simulink model "Form_Finding_Simulink"  (R2022a)
settings: Solver=ode14x  StartTime=0.0  StopTime=0.2  FixedStep=0.00005  RelTol=1e-3
values from neighbouring files (symbols this model uses):
  a_joint = 160/180*pi    (= 2.79252680319)    [Form_Finding_Activation.m]
  F_motor = F    (= 0)    [Form_Finding_Activation.m]
  g = [0;0;-9.81]    [Form_Finding_Activation.m]
  k_cable = 1200    [Form_Finding_Activation.m]
  k_joint = 35    [Form_Finding_Activation.m]
  l_cable = sqrt(6)/4*l_leg*sin(a_joint/2)*(1 - delta)    [Form_Finding_Activation.m]
  m_bar = density*(l_leg*pi*0.005^2)+ m_motor + m_battery    (= 0.662767695314)    [Form_Finding_Activation.m]
  x10_ini = x4_ini+[0 -2*bent_bar 0]    [Form_Finding_Activation.m]
  x11_ini = 2*bent_bar*rotVec([1 0 0],[0 1 0],-90-theta) + x5_ini    [Form_Finding_Activation.m]
  x12_ini = 2*bent_bar*rotVec([1 0 0],[0 1 0],-theta) + x6_ini    [Form_Finding_Activation.m]
  x1_ini = [0 0 0]    [Form_Finding_Activation.m]
  x2_ini = bent_bar*rotVec([1 0 0],[0 1 0],-theta)+ 0.5*sep*rotVec([1 0 0],[0 1 0],90-theta) + [0 sep/2 0]    [Form_Finding_Activation.m]
  x3_ini = [d6x   -sep/2         0]    [Form_Finding_Activation.m]
  x4_ini = bent_bar*rotVec([1 0 0],[0 1 0],-theta) + 0.5*sep*rotVec([1 0 0],[0 1 0],-90-theta) + [0 sep/2 0]    [Form_Finding_Activation.m]
  x5_ini = sep*rotVec([1 0 0],[0 1 0],-theta) + x3_ini    [Form_Finding_Activation.m]
  x6_ini = [0 -sep 0]    [Form_Finding_Activation.m]
  x7_ini = 2*bent_bar*rotVec([1 0 0],[0 1 0],-theta) + x1_ini    [Form_Finding_Activation.m]
  x8_ini = x2_ini + [0 -2*bent_bar 0]    [Form_Finding_Activation.m]
  x9_ini = 2*bent_bar*rotVec([1 0 0],[0 1 0],-90-theta) + x3_ini    [Form_Finding_Activation.m]
undefined symbols (not defined in the file or in its folder): l_bar
(part 2 of 2)

== matlab function Form_Finding_Simulink/6 joints/Joint bar 6--12 ==
  data: xi input; alpha output; xj input; xk input; l input; x_joint output
function [alpha, x_joint]  = angle(xi, xj, xk, l)
%% Calculating the angle
d = norm(xi - xj); % Nodal distance
mag = (l^2-2*d^2)/l^2; % Term inside the inverse cosine to calculate the angle
alpha = acos(mag); % Angle of the joint

%% Plotting the Joint
% Distance from axis
d = l/2*cos(alpha/2);

% Vectors used for determination of the normal vector
nxi = transpose(xi);
nxj = transpose(xj);
nxk = transpose(xk);

% Normal vector of a plane created by a set of 2 parallel bars
normal = cross(nxi-nxj, nxi-nxk);
N = normal/norm(normal);

% Vector along the line between bar-connected nodes
x = nxj - nxi;
X = x/norm(x);

% Vector pointing outwards 
V = rotVec(X,N,-90);

% Position vector of the joint, to be used for plotting
x_joint = transpose(d*V + (nxj+nxi)/2);

end

== matlab function Form_Finding_Simulink/24 cables/cable 1--4 ==
  data: out_i output; E_cable output; out_j output; k_cable input; l_cable input; xi input; xj input
function [out_i, E_cable, out_j]= cable(k_cable, l_cable,xi,xj)
% Node distance
dist = norm(xi-xj);

% Difference of node distance with the cable rest length
D = dist-l_cable;

% If the cable is in tension, then the force is calculated. When the cable is slack, the force is zero 
if  dist-l_cable >= 0
    D = dist-l_cable;
elseif dist-l_cable < 0
    D = 0;
end

% Forces on end nodes
out_i = k_cable*D*(xj-xi)/dist;
out_j = -k_cable*D*(xj-xi)/dist;

% Potential energy stored in the cable
E_cable = 0.5*k_cable*D^2;
end

== matlab function Form_Finding_Simulink/6 joints/Force bar 6--12 ==
  data: T input; xi input; xj input; m input; torsion_i output; torsion_j output; k_joint input; alpha input; l_bar input; a_joint input; g input
function [torsion_i, torsion_j]= Force(T, xi, xj, m, k_joint, alpha, l_bar, a_joint, g)
% Node distance
dist = norm(xj-xi);

% Force exerted by the joint at the end node. The force is zero when the
% deflection angle is larger than a_joint
if alpha < a_joint
    F_torsion = 1/2 * k_joint * (a_joint - alpha) / (cos(alpha/2)*l_bar/2);
else
    F_torsion = 0;
end

% Gravitational force:
Fg_j = m*g/2;

% Motor Force, also with the lever effect incorporated
F_motor = T/(l_bar*cos(alpha/2));

% Calculation of the two parts of the torsion
torsion_i = (F_torsion - F_motor) *(xi-xj)/dist; % % No gravity on this node because it is on the ground
torsion_j = (F_torsion - F_motor) *(xj-xi)/dist + Fg_j;

end

== matlab function Form_Finding_Simulink/12 nodes /node  4/MATLAB Function ==
  data: X input; F_out output; F_in input
function F_out = ground_constraint(X,F_in)
if X(3) <= 0 && F_in(3) < 0 
    F_out = [F_in(1);F_in(2);0];
else
    F_out = F_in;
end
end

== matlab function Form_Finding_Simulink/12 nodes /node  7/MATLAB Function ==
  data: X input; F_out output; F_in input
function F_out = ground_constraint(X,F_in)
if X(3) <= 0 && F_in(3) < 0 
    F_out = [F_in(1);F_in(2);0];
else
    F_out = F_in;
end
end

== matlab function Form_Finding_Simulink/12 nodes /node  8/MATLAB Function ==
  data: X input; F_out output; F_in input
function F_out = ground_constraint(X,F_in)
if X(3) <= 0 && F_in(3) < 0 
    F_out = [F_in(1);F_in(2);0];
else
    F_out = F_in;
end

end

== matlab function Form_Finding_Simulink/12 nodes /node  9/MATLAB Function ==
  data: X input; F_out output; F_in input
function F_out = ground_constraint(X,F_in)
if X(3) <= 0 && F_in(3) < 0 
    F_out = [F_in(1);F_in(2);0];
else
    F_out = F_in;
end
end

== matlab function Form_Finding_Simulink/12 nodes /node  10/MATLAB Function ==
  data: X input; F_out output; F_in input
function F_out = ground_constraint(X,F_in)
if X(3) <= 0 && F_in(3) < 0 
    F_out = [F_in(1);F_in(2);0];
else
    F_out = F_in;
end
end

== matlab function Form_Finding_Simulink/12 nodes /node  11/MATLAB Function ==
  data: X input; F_out output; F_in input
function F_out = ground_constraint(X,F_in)
if X(3) <= 0 && F_in(3) < 0 
    F_out = [F_in(1);F_in(2);0];
else
    F_out = F_in;
end
end

== matlab function Form_Finding_Simulink/12 nodes /node  12/MATLAB Function1 ==
  data: X input; F_out output; F_in input
function F_out = ground_constraint(X,F_in)
if X(3) <= 0 && F_in(3) < 0 
    F_out = [F_in(1);F_in(2);0];
else
    F_out = F_in;
end
end

== matlab function Form_Finding_Simulink/24 cables/cable 2--3 ==
  data: out_i output; E_cable output; out_j output; k_cable input; l_cable input; xi input; xj input
function [out_i, E_cable, out_j]= cable(k_cable, l_cable,xi,xj)
% Node distance
dist = norm(xi-xj);

% Difference of node distance with the cable rest length
D = dist-l_cable;

% If the cable is in tension, then the force is calculated. When the cable is slack, the force is zero 
if  dist-l_cable >= 0
    D = dist-l_cable;
elseif dist-l_cable < 0
    D = 0;
end

% Forces on end nodes
out_i = k_cable*D*(xj-xi)/dist;
out_j = -k_cable*D*(xj-xi)/dist;

% Potential energy stored in the cable
E_cable = 0.5*k_cable*D^2;
end

== matlab function Form_Finding_Simulink/12 nodes /node  3/node 1 constrain ==
  data: control_out output; control_in input
function control_out = node3_control(control_in)

control_out = [control_in(1);control_in(2);0];
end

== matlab function Form_Finding_Simulink/12 nodes /node 1/node 1 constrain ==
  data: control_out output; control_in input
function control_out = node1_control(control_in)

control_out = [control_in(1);control_in(2);0];
end

== matlab function Form_Finding_Simulink/6 joints/Jumping direction ==
  data: alpha_p input; l_bar input; xi input; xj input; xk input; xl input; theta output; clearance output
function [theta, clearance] = Jump_Direction(alpha_p, l_bar, xi, xj, xk, xl)
% Transposes
nxi = transpose(xi);
nxj = transpose(xj);
nxk = transpose(xk);
nxl = transpose(xl);

% Normal vector
normal1 = cross(nxi-nxj, nxi-nxk);
normal2 = cross(nxi-nxl, nxi-nxk);

% Normalized
N1 = normal1/norm(normal1);
N2 = normal2/norm(normal2);

% Caclulation of jumping direction
CosTheta = max(min(dot(N2,N1)/(norm(N2)*norm(N1)),1),-1);
theta = real(acos(CosTheta));

% Calculation of lowest joint distance to ground (leg 3)
clearance = l_bar*sin(alpha_p/2 - theta);

end
